simulink model "SixPulseRect"  (R2020a)
settings: Solver=VariableStepAuto  StartTime=0.0  StopTime=0.2  RelTol=1e-3
libraries: powerlib x17
settings Model: Creator=Matthew  LastModifiedBy=Matthew
settings DataIOCC: ReturnWorkspaceOutputs=off

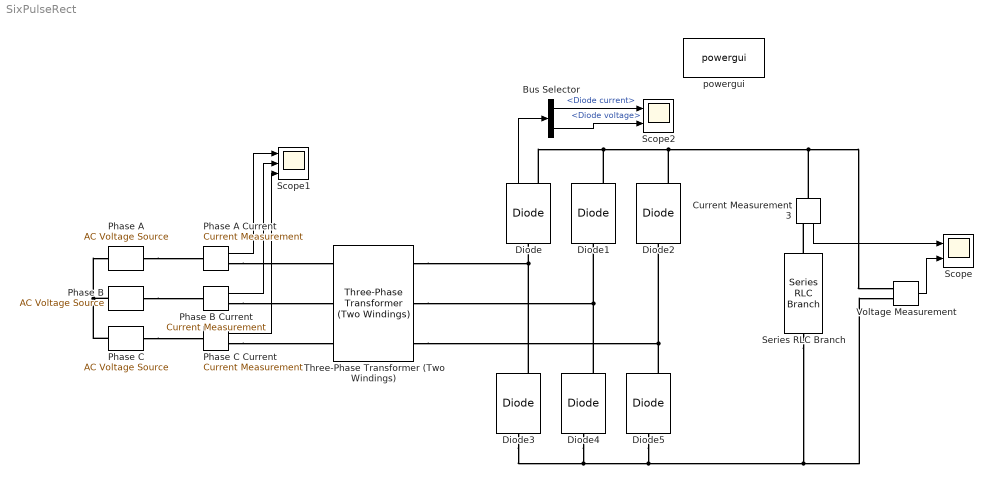
== system SixPulseRect ==
  Bus Selector : BusSelector  OutputSignals=Diode current,Diode voltage
  Current Measurement3 : powerlib/Measurements/Current Measurement  PhasorSimulation=off  OutputType=Complex  PSBequivalent=0
  Diode{,1..5} (6 alike) : powerlib/Power Electronics/Diode  Ron=0.001  Lon=0  Vf=0.8  IC=0  UseSnubber=0  Rs=500  Cs=250e-9  Measurements=on
  Phase A : powerlib/Electrical Sources/AC Voltage Source  Amplitude=(6600 * (sqrt(2))) / (sqrt(3))  Phase=0  Frequency=60  SampleTime=0  Measurements=None  BusType=swing  Pref=10e3  Qref=0  Qmin=-inf  Qmax=+inf
  Phase A Current : powerlib/Measurements/Current Measurement  PhasorSimulation=off  OutputType=Complex  PSBequivalent=0
  Phase B : powerlib/Electrical Sources/AC Voltage Source  Amplitude=(6600 * (sqrt(2))) / (sqrt(3))  Phase=120  Frequency=60  SampleTime=0  Measurements=None  BusType=swing  Pref=10e3  Qref=0  Qmin=-inf  Qmax=+inf
  "Phase B Current " : powerlib/Measurements/Current Measurement  PhasorSimulation=off  OutputType=Complex  PSBequivalent=0
  Phase C : powerlib/Electrical Sources/AC Voltage Source  Amplitude=(6600 * (sqrt(2))) / (sqrt(3))  Phase=240  Frequency=60  SampleTime=0  Measurements=None  BusType=swing  Pref=10e3  Qref=0  Qmin=-inf  Qmax=+inf
  Phase C Current : powerlib/Measurements/Current Measurement  PhasorSimulation=off  OutputType=Complex  PSBequivalent=0
  Scope : Scope  NumInputPorts=2
  Scope1 : Scope  NumInputPorts=3
  Scope2 : Scope  NumInputPorts=2
  Series RLC Branch : powerlib/Elements/Series RLC Branch  LConnTagsString=__new0  RConnTagsString=__new0  BranchType=R  Resistance=10.7973  Inductance=1e-3  SetiL0=off  InitialCurrent=0  Capacitance=1e-6  Setx0=off  InitialVoltage=0  Measurements=None
  Three-Phase Transformer (Two Windings) : powerlib/Elements/Three-Phase Transformer (Two Windings)  Winding1Connection=Y  Winding2Connection=Y  CoreType=Three single-phase transformers  SetSaturation=off  Hysteresis=off  DataFile='hysteresis'  SetInitialFlux=off  Measurements=None  UNITS=pu  NominalPower=[ 250e6 , 60 ]  Winding1=[ 6600*sqrt(3) , 0.002 , 0.08 ]  Winding2=[ 6600*sqrt(3)/2 , 0.002 , 0.08 ]  Rm=50000  Lm=500  L0=0.5  Saturation=[ 0,0 ; 0.0024,1.2 ; 1.0,1.52 ]  InitialFluxes=[ 0.8 , -0.8 , 0.7 ]  BreakLoop=off  DiscreteSolver=Trapezoidal iterative  DataType=off  TransfoNumber=1
  Voltage Measurement : powerlib/Measurements/Voltage Measurement  PhasorSimulation=off  OutputType=Complex  PSBequivalent=0
  powergui : powerlib/powergui  Priority=1  SimulationMode=Continuous  SampleTime=50e-6  frequency=60  Iterations=50  frequencyindice=60  Pbase=100e6  ErrMax=1e-4  UnitsV=kV  UnitsW=MW  buscounter=0  FunctionMessages=off  echomessages=off  EnableUseOfTLC=off  CurrentSourceSwitches=off  DisableSnubberDevices=off  DisableRonSwitches=off  DisableVfSwitches=off  DisplayEquations=off  AutomaticDiscreteSolvers=off  SolverType=Tustin/Backward Euler (TBE)  Interpol=off  ExternalGateDelay=off  methode=off  Ts=100  x0status=blocks  SPID=on  SwTol=0  HookPort=off  NonlinearTolerance=1e-4  nMaxIteration=100  ContinueOnMaxIteration=off  RestoreLinks=warning  ResistiveCurrentMeasurement=off  Frange=[0:2:500]  Ylog=off  Xlog=on  ShowGrid=off  save=off  variable=ZData  structure=ScopeData1  ZoomFFT=on  StartTime=0.1  cycles=5  DisplayStyle=1  fundamental=60  FreqAxis=off  MaxFrequency=1000  frequencyindicesteady=1  RmsSteady=1  display=off
  wires:
  Voltage Measurement/1 -> Scope/2
  Current Measurement3/1 -> Scope/1
  Phase A Current/1 -> Scope1/1
  "Phase B Current "/1 -> Scope1/2
  Phase C Current/1 -> Scope1/3
  Diode/1 -> Bus Selector/1
  Bus Selector/1 -> Scope2/1  "<Diode current>"
  Bus Selector/2 -> Scope2/2  "<Diode voltage>"
  connections:
  Diode5/RConn1 -- Three-Phase Transformer (Two Windings)/RConn3 -- Diode2/LConn1
  Diode4/RConn1 -- Three-Phase Transformer (Two Windings)/RConn2 -- Diode1/LConn1
  Diode3/RConn1 -- Three-Phase Transformer (Two Windings)/RConn1 -- Diode/LConn1
  Phase A/RConn1 -- Phase A Current/LConn1
  Phase B/RConn1 -- "Phase B Current "/LConn1
  Phase C/RConn1 -- Phase C Current/LConn1
  Phase C/LConn1 -- Phase B/LConn1 -- Phase A/LConn1
  Diode/RConn1 -- Diode1/RConn1 -- Diode2/RConn1 -- Current Measurement3/LConn1 -- Voltage Measurement/LConn1
  Diode3/LConn1 -- Diode4/LConn1 -- Diode5/LConn1 -- Voltage Measurement/LConn2 -- Series RLC Branch/RConn1
  Series RLC Branch/LConn1 -- Current Measurement3/RConn1
  Phase A Current/RConn1 -- Three-Phase Transformer (Two Windings)/LConn1
  "Phase B Current "/RConn1 -- Three-Phase Transformer (Two Windings)/LConn2
  Phase C Current/RConn1 -- Three-Phase Transformer (Two Windings)/LConn3
